simulink model "sampleModel49"  (R2021b)
settings: Solver=VariableStepAuto  StartTime=0.0  StopTime=10.0  RelTol=1e-3
libraries: simulink x2, slpidlib x1
settings Model: Creator=user  LastModifiedBy=user

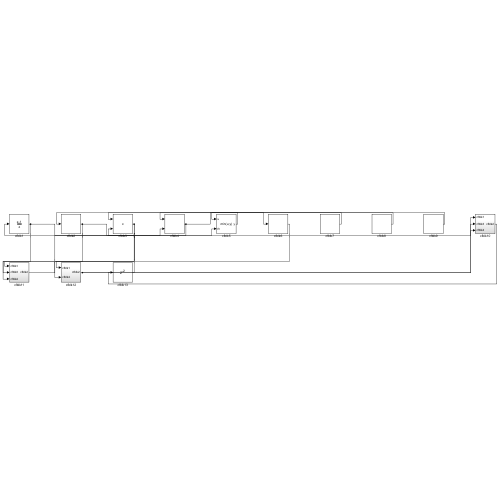
[thumbnail: Simulink's stored preview of the top-level diagram]
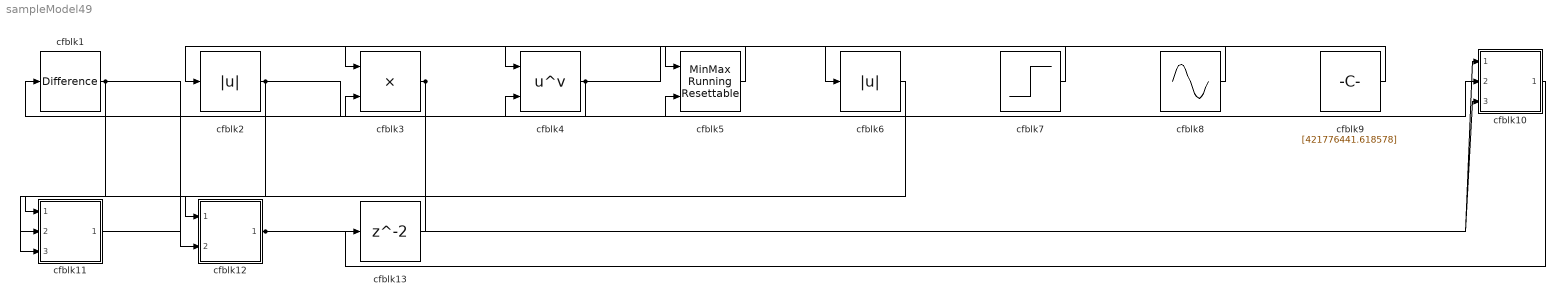
== system sampleModel49 ==
  cfblk1 : simulink/Discrete/Difference  ICPrevInput=0.0  OutMin=[]  OutMax=[]  OutDataTypeStr=Inherit: Inherit via back propagation  OutDataType=fixdt(1, 16)  OutScaling=2^-10  DoSatur=off
  cfblk10 : Subsystem
  cfblk11 : Subsystem
  cfblk12 : Subsystem
  cfblk13 : Delay  SampleTime=1
  cfblk2 : Abs
  cfblk3 : Product
  cfblk4 : Math  Operator=pow  SaturateOnIntegerOverflow=on
  cfblk5 : simulink/Math Operations/MinMax Running Resettable  Function=min  vinit=0.0
  cfblk6 : Abs
  cfblk7 : Step  Time=[9.000000]  Before=[931176241.908242]  After=[890251738.056882]  SampleTime=0
  cfblk8 : Sin  Amplitude=[-16673382.078421]  Bias=[-665482338.656915]  SampleTime=0
  cfblk9 : Constant  Value=[421776441.618578]  SampleTime=1
  wires:
  cfblk6/1 -> cfblk12/1(cfblk1)
  cfblk9/1 -> cfblk4/1
  cfblk12/1(cfblk2) -> cfblk10/1(cfblk1), cfblk10/3(cfblk4)
  cfblk8/1 -> cfblk3/1
  cfblk4/1 -> cfblk3/2, cfblk6/1
  cfblk3/1 -> cfblk11/1(cfblk1), cfblk11/2(cfblk3)
  cfblk2/1 -> cfblk4/2, cfblk12/2(cfblk4)
  cfblk11/1(cfblk2) -> cfblk10/2(cfblk3)
  cfblk7/1 -> cfblk5/1
  cfblk5/1 -> cfblk2/1
  cfblk1/1 -> cfblk5/2, cfblk11/3(cfblk4)
  cfblk10/1(cfblk2) -> cfblk13/1
  cfblk13/1 -> cfblk1/1

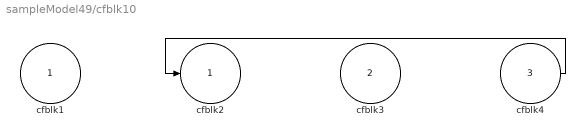
== system sampleModel49/cfblk10 ==
  cfblk1 : Inport
  cfblk3 : Inport  Port=2
  cfblk4 : Inport  Port=3
  cfblk2 : Outport
  wires:
  cfblk4/1 -> cfblk2/1

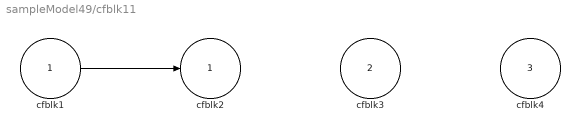
== system sampleModel49/cfblk11 ==
  cfblk1 : Inport
  cfblk3 : Inport  Port=2
  cfblk4 : Inport  Port=3
  cfblk2 : Outport
  wires:
  cfblk1/1 -> cfblk2/1

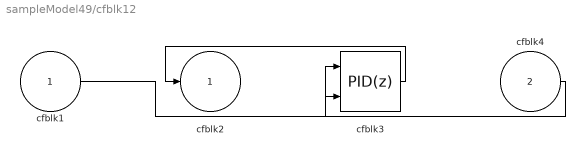
== system sampleModel49/cfblk12 ==
  cfblk1 : Inport
  cfblk4 : Inport  Port=2
  cfblk3 : slpidlib/PID Controller (2DOF)  Controller=PID  Form=Parallel  TimeDomain=Discrete-time  UseExternalTs=off  SampleTime=1  IntegratorMethod=Forward Euler  FilterMethod=Forward Euler  ControllerParametersSource=internal  P=1  I=1  D=0  UseFilter=on  N=100  b=1  c=1  TunerSelectOption=Transfer Function Based (PID Tuner App)  InitialConditionSource=internal  InitialConditionForIntegrator=0  InitialConditionForFilter=0  DifferentiatorICPrevScaledInput=0  ExternalReset=none  TrackingMode=off  Kt=1  LimitOutput=off  SatLimitsSource=internal  UpperSaturationLimit=inf  LowerSaturationLimit=-inf  LinearizeAsGain=off  AntiWindupMode=none  Kb=1  POutMin=[]  POutMax=[]  IOutMin=[]  IOutMax=[]  DOutMin=[]  DOutMax=[]  NOutMin=[]  NOutMax=[]  bOutMin=[]  bOutMax=[]  cOutMin=[]  cOutMax=[]  SumOutMin=[]  SumOutMax=[]  SaturationOutMin=[]  SaturationOutMax=[]  PParamMin=[]  PParamMax=[]  IParamMin=[]  IParamMax=[]  DParamMin=[]  DParamMax=[]  NParamMin=[]  NParamMax=[]  bParamMin=[]  bParamMax=[]  cParamMin=[]  cParamMax=[]  KbParamMin=[]  KbParamMax=[]  KtParamMin=[]  KtParamMax=[]  KbOutMin=[]  KbOutMax=[]  KtOutMin=[]  KtOutMax=[]  IntegratorOutMin=[]  IntegratorOutMax=[]  FilterOutMin=[]  FilterOutMax=[]  SumI1OutMin=[]  SumI1OutMax=[]  SumI2OutMin=[]  SumI2OutMax=[]  SumI3OutMin=[]  SumI3OutMax=[]  SumI4OutMin=[]  SumI4OutMax=[]  SumDOutMin=[]  SumDOutMax=[]  Sum1OutMin=[]  Sum1OutMax=[]  Sum2OutMin=[]  Sum2OutMax=[]  Sum3OutMin=[]  Sum3OutMax=[]  DifferentiatorOutMin=[]  DifferentiatorOutMax=[]  FilterDiffOutCoefMin=[]  FilterDiffOutCoefMax=[]  ReciprocalOutMin=[]  ReciprocalOutMax=[]  SumDenOutMin=[]  SumDenOutMax=[]  SumNumOutMin=[]  SumNumOutMax=[]  DivideOutMin=[]  DivideOutMax=[]  UdiffTsProdOutMin=[]  UdiffTsProdOutMax=[]  NTsProdOutMin=[]  NTsProdOutMax=[]  UintegralTsProdOutMin=[]  UintegralTsProdOutMax=[]  UngainTsProdOutMin=[]  UngainTsProdOutMax=[]  IntegratorContinuousStateAttributes=''  IntegratorStateMustResolveToSignalObject=off  IntegratorRTWStateStorageClass=Auto  FilterContinuousStateAttributes=''  FilterStateMustResolveToSignalObject=off  FilterRTWStateStorageClass=Auto  ParallelPVariant=InternalParameters  IdealPVariant=Disabled  IVariant=InternalParameters  DVariant=InternalParameters  bVariant=InternalParameters  cVariant=InternalParameters  IntegratorVariant=Discrete  SatVariant=Disabled  AWVariant=Passthrough  PCopyVariant=Disabled  TRVariant=Disabled  FdbkBlocksVariant=Forward  IdealPFdbkVariant=Disabled  SatFdbkVariant=Disabled  DerivativeFilterVariant=ForwardEulerFilter  NVariant=InternalParameters  NCopyVariant=Disabled  FilterICVariant=InternalICsFilter  IntegratorICVariant=InternalICs  ExternalResetVariant=Disabled  TRSumVariant=Passthrough  SumFdbkVariant=Disabled  SumVariant=Sum_PID  TsampFilterVariant=InternalTs  TsampNgainVariant=Passthrough  TsampIntegralVariant=Passthrough  ExternalSaturationOutDataTypeStr=Inherit: Same as second input
      settings: SourceProductBaseCode=SL
  cfblk2 : Outport
  wires:
  cfblk3/1 -> cfblk2/1
  cfblk1/1 -> cfblk3/1
  cfblk4/1 -> cfblk3/2
